simulink model "My_Interval_Type_2_Model"  (R2015b)
settings: Solver=FixedStepDiscrete  StartTime=0.0  StopTime=10.0  FixedStep=0.1  RelTol=1e-3
undefined symbols (not defined in the file or in its folder): evalt2
settings Model: Creator=ahmet.taskin  LastModifiedBy=ahmet.taskin

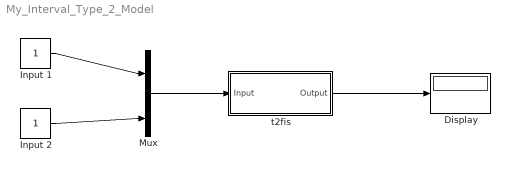
== system My_Interval_Type_2_Model ==
  Display : Display
  Input 1 : Constant  SampleTime=-1
  Input 2 : Constant  SampleTime=-1
  Mux : Mux  Inputs=2
  t2fis : Subsystem  AncestorBlock=Fuzzy_Type2_Lib/Interval Type-2 Fuzzy Logic Controller  mask(Type-2 Fuzzy Logic Controller){t2fisSim=t2fisSim}
      mask prompts: t2fisSim "t2fis name in Workspace or File Name"
      mask Display: image(imread('MemberShipMask.jpg'))
  wires:
  Input 1/1 -> Mux/1
  Input 2/1 -> Mux/2
  Mux/1 -> t2fis/1(Input)
  t2fis/1(Output) -> Display/1

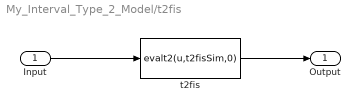
== system My_Interval_Type_2_Model/t2fis ==
  Input : Inport
  t2fis : MATLABFcn  MATLABFcn=evalt2(u,t2fisSim,0)  OutputDimensions=1
  Output : Outport
  wires:
  t2fis/1 -> Output/1
  Input/1 -> t2fis/1
